simulink model "demoACMserial"  (R2016a)
settings: Solver=FixedStepAuto  StartTime=0.0  StopTime=inf  FixedStep=1  RelTol=1e-3
undefined symbols (not defined in the file or in its folder): Green, led0
libraries: RPi x2, embdlinuxlib x1
settings Model: SimulationMode=external  Creator=user  LastModifiedBy=user
settings SolverCC: PositivePriorityOrder=on
settings OptimizationCC: OptimizeModelRefInitCode=on  LifeSpan=1  MaxStackSize=64
settings HardwareCC: ProdBitPerPointer=32  ProdLargestAtomicInteger=Long  ProdLargestAtomicFloat=Double  ProdWordSize=32  ProdHWDeviceType=ARM Compatible->ARM Cortex
settings RTWCC: SystemTargetFile=ert.tlc  HardwareBoard=Raspberry Pi  TemplateMakefile=ert_default_tmf  GenerateReport=on  Toolchain=GNU GCC Raspberry Pi  IncludeHyperlinkInReport=on  LaunchReport=on  GenerateTraceInfo=on  GenerateTraceReport=on  GenerateTraceReportSl=on  GenerateTraceReportSf=on  GenerateTraceReportEml=on
settings CodeAppCC: ForceParamTrailComments=on  IgnoreCustomStorageClasses=off  OperatorAnnotations=on  SimulinkDataObjDesc=on  SFDataObjDesc=on  MATLABFcnDesc=on  InsertBlockDesc=on  MATLABSourceComments=on
settings ERTTargetCC: SupportVariableSizeSignals=on

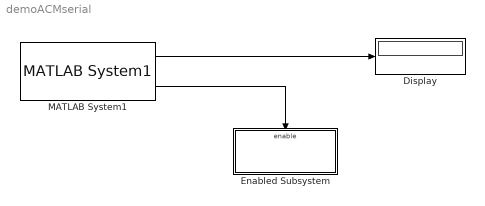
== system demoACMserial ==
  Display : Display
  Enabled Subsystem : Subsystem  TreatAsAtomicUnit=on
  MATLAB System1 : RPi/MATLAB System1  portID=0  msgLen=1  SimulateUsing=Code generation
  wires:
  MATLAB System1/1 -> Display/1
  MATLAB System1/2 -> Enabled Subsystem/Enable

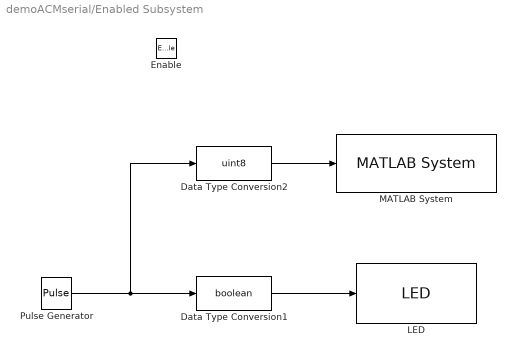
== system demoACMserial/Enabled Subsystem ==
  Enable : EnablePort
  Data Type Conversion1 : DataTypeConversion  OutDataTypeStr=boolean
  Data Type Conversion2 : DataTypeConversion  OutDataTypeStr=uint8
  LED : embdlinuxlib/LED  board=Pi 3 Model B  led=led0 (Green)  blockPlatform=Raspberry Pi
  MATLAB System : RPi/MATLAB System  portID=0  SimulateUsing=Code generation
  Pulse Generator : DiscretePulseGenerator  SampleTime=-1
  wires:
  Pulse Generator/1 -> Data Type Conversion2/1, Data Type Conversion1/1
  Data Type Conversion1/1 -> LED/1
  Data Type Conversion2/1 -> MATLAB System/1
